simulink model "identification_controllers_PID"  (R2019b)
settings: Solver=FixedStepAuto  StartTime=0.0  StopTime=inf  FixedStep=0.01  RelTol=1e-3
values from neighbouring files (symbols this model uses):
  P = double([SOL.P1;SOL.P2])    [controller_LQR_tryout.m]
  sys_dis = c2d(sys_con,Ts)    [controller_LQR_tryout.m]
  Ts = 0.02    [controller_LQR_tryout.m]
libraries: simulink x2, sldrtlib x1
settings Model: Creator=mandl  LastModifiedBy=mandl
settings SolverCC: AlgebraicLoopSolver=LineSearch

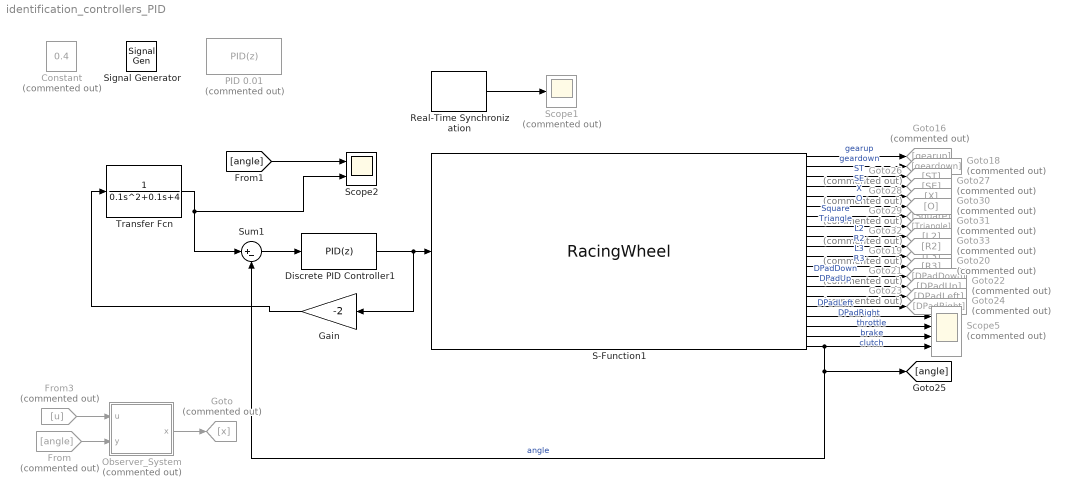
== system identification_controllers_PID ==
  Constant : Constant  Commented=on  Value=0.4
  Discrete PID Controller1 : simulink/Continuous/PID Controller  Controller=PID  Form=Parallel  TimeDomain=Discrete-time  SampleTime=0.01  IntegratorMethod=Forward Euler  FilterMethod=Forward Euler  ControllerParametersSource=internal  P=5  I=5  D=1  UseFilter=on  N=50  TunerSelectOption=Transfer Function Based (PID Tuner App)  InitialConditionSource=internal  InitialConditionForIntegrator=0  InitialConditionForFilter=0  DifferentiatorICPrevScaledInput=0  ExternalReset=none  TrackingMode=off  Kt=1  LimitOutput=on  UpperSaturationLimit=1  LowerSaturationLimit=-1  LinearizeAsGain=off  AntiWindupMode=clamping  Kb=1  POutMin=[]  POutMax=[]  IOutMin=[]  IOutMax=[]  DOutMin=[]  DOutMax=[]  NOutMin=[]  NOutMax=[]  SumOutMin=[]  SumOutMax=[]  SaturationOutMin=[]  SaturationOutMax=[]  PParamMin=[]  PParamMax=[]  IParamMin=[]  IParamMax=[]  DParamMin=[]  DParamMax=[]  NParamMin=[]  NParamMax=[]  KbParamMin=[]  KbParamMax=[]  KtParamMin=[]  KtParamMax=[]  KbOutMin=[]  KbOutMax=[]  KtOutMin=[]  KtOutMax=[]  IntegratorOutMin=[]  IntegratorOutMax=[]  FilterOutMin=[]  FilterOutMax=[]  SumI1OutMin=[]  SumI1OutMax=[]  SumI2OutMin=[]  SumI2OutMax=[]  SumI3OutMin=[]  SumI3OutMax=[]  SumI4OutMin=[]  SumI4OutMax=[]  SumDOutMin=[]  SumDOutMax=[]  DifferentiatorOutMin=[]  DifferentiatorOutMax=[]  FilterDiffOutCoefMin=[]  FilterDiffOutCoefMax=[]  ReciprocalOutMin=[]  ReciprocalOutMax=[]  SumDenOutMin=[]  SumDenOutMax=[]  SumNumOutMin=[]  SumNumOutMax=[]  DivideOutMin=[]  DivideOutMax=[]  IntegratorContinuousStateAttributes=''  IntegratorStateMustResolveToSignalObject=off  IntegratorRTWStateStorageClass=Auto  FilterContinuousStateAttributes=''  FilterStateMustResolveToSignalObject=off  FilterRTWStateStorageClass=Auto  ParallelPVariant=InternalParameters  IdealPVariant=Disabled  IVariant=InternalParameters  DVariant=InternalParameters  IntegratorVariant=Discrete  SatVariant=Enabled  AWVariant=DiscClampingParallel  PCopyVariant=Disabled  TRVariant=Disabled  FdbkBlocksVariant=Forward  IdealPFdbkVariant=Disabled  SatFdbkVariant=Disabled  DerivativeFilterVariant=ForwardEulerFilter  NVariant=InternalParameters  NCopyVariant=Disabled  FilterICVariant=InternalICsFilter  IntegratorICVariant=InternalICs  ExternalResetVariant=Disabled  TRSumVariant=Passthrough  SumFdbkVariant=Disabled  SumVariant=Sum_PID
  From : From  Commented=on  GotoTag=angle
  From3 : From  Commented=on  GotoTag=u
  Gain : Gain  Gain=-2
  Goto : Goto  Commented=on  GotoTag=x
  Goto16 : Goto  Commented=on  GotoTag=gearup
  Goto18 : Goto  Commented=on  GotoTag=geardown
  Goto19 : Goto  Commented=on  GotoTag=L3
  Goto20 : Goto  Commented=on  GotoTag=R3
  Goto21 : Goto  Commented=on  GotoTag=DPadDown
  Goto22 : Goto  Commented=on  GotoTag=DPadUp
  Goto23 : Goto  Commented=on  GotoTag=DPadLeft
  Goto24 : Goto  Commented=on  GotoTag=DPadRight
  Goto26 : Goto  Commented=on  GotoTag=ST
  Goto27 : Goto  Commented=on  GotoTag=SE
  Goto28 : Goto  Commented=on  GotoTag=X
  Goto29 : Goto  Commented=on  GotoTag=Square
  Goto30 : Goto  Commented=on  GotoTag=O
  Goto31 : Goto  Commented=on  GotoTag=Triangle
  Goto32 : Goto  Commented=on  GotoTag=L2
  Goto33 : Goto  Commented=on  GotoTag=R2
  Observer_System : Subsystem  Commented=on
  PID 0.01 : simulink/Continuous/PID Controller  Commented=on  Controller=PID  Form=Parallel  TimeDomain=Discrete-time  SampleTime=0.01  IntegratorMethod=Forward Euler  FilterMethod=Forward Euler  ControllerParametersSource=internal  P=5  I=5  D=1  UseFilter=on  N=50  TunerSelectOption=Transfer Function Based (PID Tuner App)  InitialConditionSource=internal  InitialConditionForIntegrator=0  InitialConditionForFilter=0  DifferentiatorICPrevScaledInput=0  ExternalReset=none  TrackingMode=off  Kt=1  LimitOutput=on  UpperSaturationLimit=1  LowerSaturationLimit=-1  LinearizeAsGain=off  AntiWindupMode=clamping  Kb=1  POutMin=[]  POutMax=[]  IOutMin=[]  IOutMax=[]  DOutMin=[]  DOutMax=[]  NOutMin=[]  NOutMax=[]  SumOutMin=[]  SumOutMax=[]  SaturationOutMin=[]  SaturationOutMax=[]  PParamMin=[]  PParamMax=[]  IParamMin=[]  IParamMax=[]  DParamMin=[]  DParamMax=[]  NParamMin=[]  NParamMax=[]  KbParamMin=[]  KbParamMax=[]  KtParamMin=[]  KtParamMax=[]  KbOutMin=[]  KbOutMax=[]  KtOutMin=[]  KtOutMax=[]  IntegratorOutMin=[]  IntegratorOutMax=[]  FilterOutMin=[]  FilterOutMax=[]  SumI1OutMin=[]  SumI1OutMax=[]  SumI2OutMin=[]  SumI2OutMax=[]  SumI3OutMin=[]  SumI3OutMax=[]  SumI4OutMin=[]  SumI4OutMax=[]  SumDOutMin=[]  SumDOutMax=[]  DifferentiatorOutMin=[]  DifferentiatorOutMax=[]  FilterDiffOutCoefMin=[]  FilterDiffOutCoefMax=[]  ReciprocalOutMin=[]  ReciprocalOutMax=[]  SumDenOutMin=[]  SumDenOutMax=[]  SumNumOutMin=[]  SumNumOutMax=[]  DivideOutMin=[]  DivideOutMax=[]  IntegratorContinuousStateAttributes=''  IntegratorStateMustResolveToSignalObject=off  IntegratorRTWStateStorageClass=Auto  FilterContinuousStateAttributes=''  FilterStateMustResolveToSignalObject=off  FilterRTWStateStorageClass=Auto  ParallelPVariant=InternalParameters  IdealPVariant=Disabled  IVariant=InternalParameters  DVariant=InternalParameters  IntegratorVariant=Discrete  SatVariant=Enabled  AWVariant=DiscClampingParallel  PCopyVariant=Disabled  TRVariant=Disabled  FdbkBlocksVariant=Forward  IdealPFdbkVariant=Disabled  SatFdbkVariant=Disabled  DerivativeFilterVariant=ForwardEulerFilter  NVariant=InternalParameters  NCopyVariant=Disabled  FilterICVariant=InternalICsFilter  IntegratorICVariant=InternalICs  ExternalResetVariant=Disabled  TRSumVariant=Passthrough  SumFdbkVariant=Disabled  SumVariant=Sum_PID
  Real-Time Synchronization : sldrtlib/Real-Time Synchronization  SampleTime=0.01  MaxMissedTicks=inf  ShowMissedTicks=on  YieldWhenWaiting=off
  S-Function1 : S-Function  FunctionName=RacingWheel  Parameters=Ts_FF  SFunctionModules=RacingWheel_wrapper  SFunctionDeploymentMode=off  EnableBusSupport=off  mask(Racing Wheel with Force Feedback){Ts_FF=0.01}
      mask prompts: Ts_FF "Constant Force-Feedback Sample Time"
      mask help: Interacts with the windows gaming API from UWP. The force feedback effect is constant over the user defined sampling time below.
      mask init:
      | val = [[.9  0.75 0.75 1 1 .9 .9 1]',[1 1 0.75 0.75 .9 .9 1 .9]'];try , sys = get_param(gcb,'SfunBuilderFcnName');if isempty(sys), sys = get_param(gcb,'FunctionName'); end,catch, sys = get_param(gcb,'FunctionName'); end
      mask Display:
      | plot(val(:,1),val(:,2)),disp(sys),
      | image('icon.png'),
      | port_label('input',1,'FF'),
      | port_label('output',1,'gearup'),
      | port_label('output',2,'geardown'),
      | port_label('output',3,'ST'),
      | port_label('output',4,'SE'),
      | port_label('output',5,'X'),
      | port_label('output',6,'O'),
      | port_label('output',7,'Square'),
      | port_label('output',8,'Triangle'),
      | port_label('output',9,'L2'),
      | port_label('output',10,'R2'),
      | port_label('output',11,'L3'),
      | port_label('output',12,'R3'),
      | port_label('output',13,'DPadDown'),
      | port_label('output',14,'DPadUp'),
      | port_label('output',15,'DPadLeft'),
      | port_label('output',16,'DPadRight'),
      | port_label('output',17,'throttle'),
      | port_label('output',18,'brake'),
      | port_label('output',19,'clutch'),
      | port_label('output',20,'angle')
  Scope1 : Scope  Commented=on
  Scope2 : Scope  NumInputPorts=2
  Scope5 : Scope  Commented=on  NumInputPorts=4
  Signal Generator : SignalGenerator  Amplitude=0.9  Frequency=0.3
  Sum1 : Sum  Inputs=|+-
  Transfer Fcn : TransferFcn  Denominator=[0.1 0.1 4]
  wires:
  Real-Time Synchronization/1 -> Scope1/1
  S-Function1/4 -> Goto27/1  "SE"
  S-Function1/17 -> Scope5/1  "throttle"
  S-Function1/5 -> Goto28/1  "X"
  S-Function1/13 -> Goto21/1  "DPadDown"
  Sum1/1 -> Discrete PID Controller1/1
  S-Function1/8 -> Goto31/1  "Triangle"
  S-Function1/11 -> Goto19/1  "L3"
  S-Function1/10 -> Goto33/1  "R2"
  S-Function1/1 -> Goto16/1  "gearup"
  S-Function1/18 -> Scope5/2  "brake"
  S-Function1/14 -> Goto22/1  "DPadUp"
  S-Function1/3 -> Goto26/1  "ST"
  S-Function1/6 -> Goto30/1  "O"
  S-Function1/7 -> Goto29/1  "Square"
  S-Function1/15 -> Goto23/1  "DPadLeft"
  S-Function1/9 -> Goto32/1  "L2"
  S-Function1/12 -> Goto20/1  "R3"
  S-Function1/2 -> Goto18/1  "geardown"
  Transfer Fcn/1 -> Scope2/2, Sum1/1
  S-Function1/19 -> Scope5/3  "clutch"
  S-Function1/16 -> Goto24/1  "DPadRight"
  S-Function1/20 -> Scope5/4, Sum1/2, [angle]  "angle"
  Observer_System/1(x) -> Goto/1
  From/1 -> Observer_System/2(y)
  From3/1 -> Observer_System/1(u)
  Discrete PID Controller1/1 -> Gain/1, S-Function1/1
  Gain/1 -> Transfer Fcn/1
  [angle] -> Scope2/1

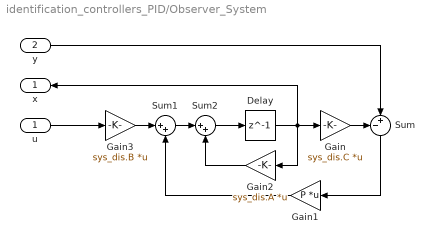
== system identification_controllers_PID/Observer_System ==
  u : Inport
  y : Inport  Port=2
  Delay : Delay  DelayLength=1  InitialCondition=[0,0]  SampleTime=Ts
  Gain : Gain  Gain=sys_dis.C  Multiplication=Matrix(K*u)
  Gain1 : Gain  Gain=P  Multiplication=Matrix(K*u)
  Gain2 : Gain  Gain=sys_dis.A  Multiplication=Matrix(K*u)
  Gain3 : Gain  Gain=sys_dis.B  Multiplication=Matrix(K*u)
  Sum : Sum  Inputs=-+|
  Sum1 : Sum  Inputs=|++
  Sum2 : Sum  Inputs=|++
  x : Outport
  wires:
  Sum/1 -> Gain1/1
  u/1 -> Gain3/1
  Gain/1 -> Sum/1
  Gain1/1 -> Sum1/2
  Sum1/1 -> Sum2/1
  Delay/1 -> x/1, Gain2/1, Gain/1
  Sum2/1 -> Delay/1
  Gain2/1 -> Sum2/2
  Gain3/1 -> Sum1/1
  y/1 -> Sum/2
